simulink model "completed_microinverter_setup"  (R2022a)
settings: Solver=FixedStepDiscrete  StartTime=0.0  StopTime=2  FixedStep=Ts  RelTol=1e-3
InitFcn:
  | Ts=1e-6;
  | Tcs=1e-4;
values from neighbouring files (symbols this model uses):
  C1_filter = 2e-6    (= 2e-06)    [q4.m]
  C_filter = 100e-6    (= 0.0001)    [q1.m]    (also in q2.m; q4.m = 2e-06)
  f_center = 50    [q4.m]
  F_switch = 1e3    (= 1000)    [q1.m]
  Ki_current = L_filter*Wn^2    (= 15791.3670417)    [q1.m]    (also in q2.m = 63165.468167; q4.m = 493.480220054)
  Ki_pll = (Wn^2) / A    (= 394784.176044)    [q1.m]    (also in q4.m = 1579136.70417)
  Ki_power = 100    [q4.m]
  Ki_voltage = C_filter*Wn^2    (= 3.55305758439)    [q1.m]    (also in q4.m = 0.0710611516878)
  Kp_current = 2*L_filter*DF*Wn    (= 110.584061406)    [q1.m]    (also in q2.m = 71.0753921948; q4.m = 5.49778714378)
  Kp_pll = 2*DF / sqrt(A/Ki_pll)    [q1.m]    (also in q4.m = 2*DF / sqrt(1/Ki_pll))
  Kp_power = 0    [q4.m]
  Kp_voltage = 2*C_filter*DF*Wn    (= 0.0565486677646)    [q1.m]    (also in q4.m = 0.00791681348705)
  L1_filter = 1.5e-3    (= 0.0015)    [q4.m]
  L2_filter = 1.0e-3    (= 0.001)    [q4.m]
  L_filter = 40e-3    (= 0.04)    [q1.m]    (also in q2.m; q4.m = 0.00125)
  L_load = sqrt((R_load * V_rms^2)/P_load - R_load^2) / w    [q1.m]    (also in q4.m)
  R_load = (V_rms^2) * (pf_load^2) / P_load    (= 43.32)    [q1.m]    (also in q4.m)
  Rd_filter = 0.2    [q4.m]
  Tes = 20*Ts    (= 2e-05)    [q1.m]    (also in q4.m)
  V_dc = sqrt(2) * sqrt(3) * V_rms    [q1.m]    (also in q4.m = V_rms * sqrt(3) * sqrt(2))
undefined symbols (not defined in the file or in its folder): DiscIntNeverNeededParam
libraries: ee_lib x111, nesl_utility x28, fl_lib x23, spsabctodq0Lib x11, dspindex x3, spsTriangleGeneratorLib x2, spsdq0toabcLib x2
(part 2 of 4)

== system completed_microinverter_setup/Transmission line series impedance ==
  Inductor1 : ee_lib/Passive/Inductor  l=L H  enable_L_tol=0  L_tol=20  tol_distribution=1  nSigma=4  r=0 Ohm  g=1e-9 1/Ohm  enable_operating_limits=0  operating_limit_action=2  max_working_current=1 A  power_rating=1 W  enable_faults=0  fault_action=1  lambdaPercent=50  k_faulted=0.9999  turnsShort=0  openCct=0  groundShort=0  groundShortG=0 1/Ohm  tau_fault=1e-3 s  enable_temporal_fault=0  t_fault=1 s  enable_behavioral_fault=0  max_permissible_voltage=100 V  n_fail_on_voltage=1  max_permissible_current=1 A  t_fail_on_current=1 s  i_L_specify=off  i_L_priority=High  i_L=0 A  i_L_nominal_specify=off  i_L_nominal_unit=A  i_L_nominal_value=1
  Inductor2 : ee_lib/Passive/Inductor  l=L H  enable_L_tol=0  L_tol=20  tol_distribution=1  nSigma=4  r=0 Ohm  g=1e-9 1/Ohm  enable_operating_limits=0  operating_limit_action=2  max_working_current=1 A  power_rating=1 W  enable_faults=0  fault_action=1  lambdaPercent=50  k_faulted=0.9999  turnsShort=0  openCct=0  groundShort=0  groundShortG=0 1/Ohm  tau_fault=1e-3 s  enable_temporal_fault=0  t_fault=1 s  enable_behavioral_fault=0  max_permissible_voltage=100 V  n_fail_on_voltage=1  max_permissible_current=1 A  t_fail_on_current=1 s  i_L_specify=off  i_L_priority=High  i_L=0 A  i_L_nominal_specify=off  i_L_nominal_unit=A  i_L_nominal_value=1
  Inductor3 : ee_lib/Passive/Inductor  l=L H  enable_L_tol=0  L_tol=20  tol_distribution=1  nSigma=4  r=0 Ohm  g=1e-9 1/Ohm  enable_operating_limits=0  operating_limit_action=2  max_working_current=1 A  power_rating=1 W  enable_faults=0  fault_action=1  lambdaPercent=50  k_faulted=0.9999  turnsShort=0  openCct=0  groundShort=0  groundShortG=0 1/Ohm  tau_fault=1e-3 s  enable_temporal_fault=0  t_fault=1 s  enable_behavioral_fault=0  max_permissible_voltage=100 V  n_fail_on_voltage=1  max_permissible_current=1 A  t_fail_on_current=1 s  i_L_specify=off  i_L_priority=High  i_L=0 A  i_L_nominal_specify=off  i_L_nominal_unit=A  i_L_nominal_value=1
  Phase Splitter : ee_lib/Connectors & References/Phase Splitter
      settings: SourceProductBaseCode=PS
  Phase Splitter1 : ee_lib/Connectors & References/Phase Splitter
      settings: SourceProductBaseCode=PS
  Resistor : ee_lib/Passive/Resistor  R=R Ohm  enable_R_tol=0  R_tol=5  tol_distribution=1  nSigma=4  enable_operating_limits=0  operating_limit_action=2  max_working_voltage=100 V  power_rating=1 W  enable_faults=0  fault_action=1  R_faulted=inf Ohm  enable_temporal_fault=0  t_fault=1 s  enable_behavioral_fault=0  max_permissible_current=1 A  t_fail_on_current=1 s  noise_mode=0  sample_time=1e-3 s  repeatability=1  auto_seed=676943032  user_seed=0  Tdevice=25 degC  power_derating_T1=70 degC  power_derating_T2=155 degC  operating_temperature_range_vec=[-50, 150] degC  alpha=3.93e-3 1/K  Tmeas=25 degC  thermal_mass=100 J/K  temperature_specify=off  temperature_priority=High  temperature=298.15 K  temperature_nominal_specify=off  temperature_nominal_unit=K  temperature_nominal_value=1
  Resistor1 : ee_lib/Passive/Resistor  R=R Ohm  enable_R_tol=0  R_tol=5  tol_distribution=1  nSigma=4  enable_operating_limits=0  operating_limit_action=2  max_working_voltage=100 V  power_rating=1 W  enable_faults=0  fault_action=1  R_faulted=inf Ohm  enable_temporal_fault=0  t_fault=1 s  enable_behavioral_fault=0  max_permissible_current=1 A  t_fail_on_current=1 s  noise_mode=0  sample_time=1e-3 s  repeatability=1  auto_seed=4168664255  user_seed=0  Tdevice=25 degC  power_derating_T1=70 degC  power_derating_T2=155 degC  operating_temperature_range_vec=[-50, 150] degC  alpha=3.93e-3 1/K  Tmeas=25 degC  thermal_mass=100 J/K  temperature_specify=off  temperature_priority=High  temperature=298.15 K  temperature_nominal_specify=off  temperature_nominal_unit=K  temperature_nominal_value=1
  Resistor2 : ee_lib/Passive/Resistor  R=R Ohm  enable_R_tol=0  R_tol=5  tol_distribution=1  nSigma=4  enable_operating_limits=0  operating_limit_action=2  max_working_voltage=100 V  power_rating=1 W  enable_faults=0  fault_action=1  R_faulted=inf Ohm  enable_temporal_fault=0  t_fault=1 s  enable_behavioral_fault=0  max_permissible_current=1 A  t_fail_on_current=1 s  noise_mode=0  sample_time=1e-3 s  repeatability=1  auto_seed=4111000739  user_seed=0  Tdevice=25 degC  power_derating_T1=70 degC  power_derating_T2=155 degC  operating_temperature_range_vec=[-50, 150] degC  alpha=3.93e-3 1/K  Tmeas=25 degC  thermal_mass=100 J/K  temperature_specify=off  temperature_priority=High  temperature=298.15 K  temperature_nominal_specify=off  temperature_nominal_unit=K  temperature_nominal_value=1
  V_in : PMIOPort  Side=Left
  V_out : PMIOPort  Port=2  Side=Right
  connections:
  Phase Splitter1/RConn1 -- Inductor3/LConn1
  Inductor2/LConn1 -- Phase Splitter1/RConn3
  Inductor1/LConn1 -- Phase Splitter1/RConn2
  V_in/RConn1 -- Phase Splitter1/LConn1
  Resistor1/LConn1 -- Inductor1/RConn1
  Phase Splitter/RConn3 -- Resistor2/RConn1
  Phase Splitter/RConn1 -- Resistor/RConn1
  V_out/RConn1 -- Phase Splitter/LConn1
  Resistor/LConn1 -- Inductor3/RConn1
  Phase Splitter/RConn2 -- Resistor1/RConn1
  Resistor2/LConn1 -- Inductor2/RConn1

== system completed_microinverter_setup/Calculate PQ of output/Subsystem ==
  Vdq0 : Inport
  Constant : Constant
  Demux : Demux  Outputs=3
  Divide : Product  Inputs=*/
  Gain : Gain  Gain=-1
  Matrix Concatenate : Concatenate  Mode=Multidimensional array
  Matrix Concatenate1 : Concatenate  Mode=Multidimensional array  ConcatenateDimension=2
  Mux : Mux
  Reshape : Reshape  OutputDimensionality=Customize  OutputDimensions=[2,2]
  Sqrt1 : Sqrt
  Sqrt2 : Sqrt
  Square1 : Math  Operator=square
  Subtract : Sum  Inputs=+-
  Sum : Sum  Inputs=|++
  Terminator : Terminator
  Zero : Constant  Value=zeros(1,2)  VectorParams1D=off  OutDataTypeStr=Inherit: Inherit via back propagation
  Zero1 : Constant  Value=zeros(3,1)  VectorParams1D=off  OutDataTypeStr=Inherit: Inherit via back propagation
  Rotation Matrix : Outport
  wires:
  Vdq0/1 -> Square1/1
  Demux/1 -> Divide/1, Sum/1  "Vd^2"
  Reshape/1 -> Matrix Concatenate/1
  Gain/1 -> Mux/2
  Divide/1 -> Subtract/2, Sqrt1/1  "Vd^2 / (Vd^2 + Vq^2)"
  Sqrt2/1 -> Mux/3, Gain/1  "sin(theta)"
  Subtract/1 -> Sqrt2/1
  Demux/3 -> Terminator/1
  Square1/1 -> Demux/1
  Mux/1 -> Reshape/1
  Demux/2 -> Sum/2  "Vq^2"
  Constant/1 -> Subtract/1
  Sqrt1/1 -> Mux/4, Mux/1  "cos(theta)"
  Sum/1 -> Divide/2
  Zero/1 -> Matrix Concatenate/2
  Zero1/1 -> Matrix Concatenate1/2
  Matrix Concatenate/1 -> Matrix Concatenate1/1
  Matrix Concatenate1/1 -> Rotation Matrix/1

== system completed_microinverter_setup/Grid Feeding//Forming Inverter 1/3 Phase Grid Sensor ==
  Neutral Port (Three-Phase) : ee_lib/Connectors & References/Neutral Port (Three-Phase)  G_parasitic=1e-12 1/Ohm
      settings: SourceProductBaseCode=PS  InternalSimscapePortConfiguration="{\"Bottom\":[],\"Left\":[{\"id\":\"N\",\"label\":\"~\",\"type\":\"foundation.electrical.three_phase\"}],\"Right\":[{\"id\":\"n\",\"label\":\"n\",\"type\":\"foundation.electrical.electrical\"}],\"Top\":[]}"
  PS-Simulink Converter : nesl_utility/PS-Simulink Converter  PhysicalDomain=network_engine_domain  SubClassName=ps_output  LeftPortType=input  RightPortType=output  PseudoPeriodic=off  Frequencies=[]  VectorFormat=inherit  Unit=inherit  AffineConversion=off
      settings: SourceProductBaseCode=SS,PW,VE
  Phase Splitter1 : ee_lib/Connectors & References/Phase Splitter
      settings: SourceProductBaseCode=PS
  Phase Voltage Sensor (Three-Phase) : ee_lib/Sensors & Transducers/Phase Voltage Sensor (Three-Phase)
      settings: SourceProductBaseCode=PS
  Resistor : ee_lib/Passive/Resistor  R=R Ohm  enable_R_tol=0  R_tol=5  tol_distribution=1  nSigma=4  enable_operating_limits=0  operating_limit_action=2  max_working_voltage=100 V  power_rating=1 W  enable_faults=0  fault_action=1  R_faulted=inf Ohm  enable_temporal_fault=0  t_fault=1 s  enable_behavioral_fault=0  max_permissible_current=1 A  t_fail_on_current=1 s  noise_mode=0  sample_time=1e-3 s  repeatability=1  auto_seed=2715962282  user_seed=0  Tdevice=25 degC  power_derating_T1=70 degC  power_derating_T2=155 degC  operating_temperature_range_vec=[-50, 150] degC  alpha=3.93e-3 1/K  Tmeas=25 degC  thermal_mass=100 J/K  temperature_specify=off  temperature_priority=High  temperature=298.15 K  temperature_nominal_specify=off  temperature_nominal_unit=K  temperature_nominal_value=1
  Resistor1 : ee_lib/Passive/Resistor  R=R Ohm  enable_R_tol=0  R_tol=5  tol_distribution=1  nSigma=4  enable_operating_limits=0  operating_limit_action=2  max_working_voltage=100 V  power_rating=1 W  enable_faults=0  fault_action=1  R_faulted=inf Ohm  enable_temporal_fault=0  t_fault=1 s  enable_behavioral_fault=0  max_permissible_current=1 A  t_fail_on_current=1 s  noise_mode=0  sample_time=1e-3 s  repeatability=1  auto_seed=418932850  user_seed=0  Tdevice=25 degC  power_derating_T1=70 degC  power_derating_T2=155 degC  operating_temperature_range_vec=[-50, 150] degC  alpha=3.93e-3 1/K  Tmeas=25 degC  thermal_mass=100 J/K  temperature_specify=off  temperature_priority=High  temperature=298.15 K  temperature_nominal_specify=off  temperature_nominal_unit=K  temperature_nominal_value=1
  Resistor2 : ee_lib/Passive/Resistor  R=R Ohm  enable_R_tol=0  R_tol=5  tol_distribution=1  nSigma=4  enable_operating_limits=0  operating_limit_action=2  max_working_voltage=100 V  power_rating=1 W  enable_faults=0  fault_action=1  R_faulted=inf Ohm  enable_temporal_fault=0  t_fault=1 s  enable_behavioral_fault=0  max_permissible_current=1 A  t_fail_on_current=1 s  noise_mode=0  sample_time=1e-3 s  repeatability=1  auto_seed=1196140742  user_seed=0  Tdevice=25 degC  power_derating_T1=70 degC  power_derating_T2=155 degC  operating_temperature_range_vec=[-50, 150] degC  alpha=3.93e-3 1/K  Tmeas=25 degC  thermal_mass=100 J/K  temperature_specify=off  temperature_priority=High  temperature=298.15 K  temperature_nominal_specify=off  temperature_nominal_unit=K  temperature_nominal_value=1
  V_abc : PMIOPort  Side=Left
  V_abc_sense : Outport
  wires:
  PS-Simulink Converter/1 -> V_abc_sense/1
  connections:
  Resistor2/LConn1 -- Phase Splitter1/RConn3
  Resistor/RConn1 -- Neutral Port (Three-Phase)/RConn1 -- Resistor2/RConn1 -- Resistor1/RConn1
  Phase Splitter1/RConn2 -- Resistor1/LConn1
  Phase Splitter1/RConn1 -- Resistor/LConn1
  V_abc/RConn1 -- Phase Voltage Sensor (Three-Phase)/LConn1 -- Phase Splitter1/LConn1
  Phase Voltage Sensor (Three-Phase)/RConn2 -- Neutral Port (Three-Phase)/LConn1
  PS-Simulink Converter/LConn1 -- Phase Voltage Sensor (Three-Phase)/RConn1

== system completed_microinverter_setup/Grid Feeding//Forming Inverter 1/Calculate PQ of output ==
  note: Reorient Vdq0 so that Uq = 0, Ud = defined
  Vdq0 : Inport
  Idq0 : Inport  Port=2
  Atan2 : Trigonometry  Operator=atan2
  Cos : Trigonometry  Operator=cos
  Demux : Demux  Outputs=3
  Demux1 : Demux  Outputs=2
  Gain2 : Gain  Gain=3/2
  MatrixMultiply1 : Product  Multiplication=Matrix(*)
  MatrixMultiply2 : Product  Multiplication=Matrix(*)
  Mux : Mux
  Product : Product
  Product2 : Product
  Selector : Selector  InputPortWidth=3  IndexOptions=Index vector (dialog)  Indices=[1 2]  OutputSizes=1
  Selector1 : Selector  InputPortWidth=3  IndexOptions=Index vector (dialog)  Indices=[1]  OutputSizes=1
  Sign : Signum
  Sqrt : Sqrt
  Square : Math  Operator=square
  Subsystem : Subsystem
  Sum of Elements : Sum  Inputs=+
  Terminator : Terminator
  PQ Stats : Outport
  wires:
  Product2/1 -> Gain2/1
  Square/1 -> Sum of Elements/1
  Gain2/1 -> Demux/1, Selector/1
  Sum of Elements/1 -> Sqrt/1
  Selector/1 -> Square/1, Demux1/1
  Vdq0/1 -> MatrixMultiply1/2, Subsystem/1(Vdq0)
  Subsystem/1(Rotation Matrix) -> MatrixMultiply2/1, MatrixMultiply1/1
  Idq0/1 -> MatrixMultiply2/2
  MatrixMultiply1/1 -> Selector1/1
  MatrixMultiply2/1 -> Product2/2
  Demux/3 -> Terminator/1
  Demux/2 -> Atan2/1  "Q"
  Demux/1 -> Atan2/2  "P"
  Atan2/1 -> Cos/1
  Demux1/1 -> Mux/1  "P"
  Demux1/2 -> Sign/1, Mux/2  "Q"
  Sqrt/1 -> Mux/3  "|S|"
  Product/1 -> Mux/4  "pf"
  Mux/1 -> PQ Stats/1
  Selector1/1 -> Product2/1
  Sign/1 -> Product/1
  Cos/1 -> Product/2  "pf"

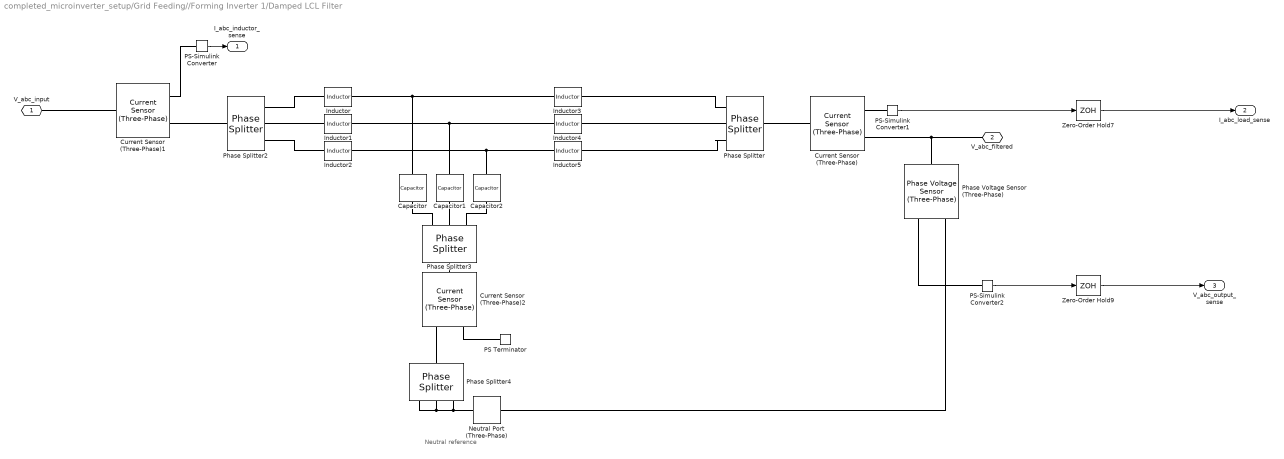
== system completed_microinverter_setup/Grid Feeding//Forming Inverter 1/Damped LCL Filter ==
  note: Neutral reference
  Capacitor : fl_lib/Electrical/Electrical Elements/Capacitor  c=C F  r=Rd Ohm  g=0 1/Ohm  i_specify=off  i_priority=None  i=0 A  i_nominal_specify=off  i_nominal_unit=A  i_nominal_value=1  v_specify=off  v_priority=None  v=0 V  v_nominal_specify=off  v_nominal_unit=V  v_nominal_value=1  vc_specify=off  vc_priority=High  vc=0 V  vc_nominal_specify=off  vc_nominal_unit=V  vc_nominal_value=1
      settings: SourceProductBaseCode=PW,SS,VE
  Capacitor1 : fl_lib/Electrical/Electrical Elements/Capacitor  c=C F  r=Rd Ohm  g=0 1/Ohm  i_specify=off  i_priority=None  i=0 A  i_nominal_specify=off  i_nominal_unit=A  i_nominal_value=1  v_specify=off  v_priority=None  v=0 V  v_nominal_specify=off  v_nominal_unit=V  v_nominal_value=1  vc_specify=off  vc_priority=High  vc=0 V  vc_nominal_specify=off  vc_nominal_unit=V  vc_nominal_value=1
      settings: SourceProductBaseCode=PW,SS,VE
  Capacitor2 : fl_lib/Electrical/Electrical Elements/Capacitor  c=C F  r=Rd Ohm  g=0 1/Ohm  i_specify=off  i_priority=None  i=0 A  i_nominal_specify=off  i_nominal_unit=A  i_nominal_value=1  v_specify=off  v_priority=None  v=0 V  v_nominal_specify=off  v_nominal_unit=V  v_nominal_value=1  vc_specify=off  vc_priority=High  vc=0 V  vc_nominal_specify=off  vc_nominal_unit=V  vc_nominal_value=1
      settings: SourceProductBaseCode=PW,SS,VE
  Current Sensor (Three-Phase) : ee_lib/Sensors & Transducers/Current Sensor (Three-Phase)
  Current Sensor (Three-Phase)1 : ee_lib/Sensors & Transducers/Current Sensor (Three-Phase)
  Current Sensor (Three-Phase)2 : ee_lib/Sensors & Transducers/Current Sensor (Three-Phase)
  Inductor : ee_lib/Passive/Inductor  l=L1 H  enable_L_tol=0  L_tol=20  tol_distribution=1  nSigma=4  r=0 Ohm  g=1e-9 1/Ohm  enable_operating_limits=0  operating_limit_action=2  max_working_current=1 A  power_rating=1 W  enable_faults=0  fault_action=1  lambdaPercent=50  k_faulted=0.9999  turnsShort=0  openCct=0  groundShort=0  groundShortG=0 1/Ohm  tau_fault=1e-3 s  enable_temporal_fault=0  t_fault=1 s  enable_behavioral_fault=0  max_permissible_voltage=100 V  n_fail_on_voltage=1  max_permissible_current=1 A  t_fail_on_current=1 s  i_L_specify=off  i_L_priority=High  i_L=0 A  i_L_nominal_specify=off  i_L_nominal_unit=A  i_L_nominal_value=1
  Inductor1 : ee_lib/Passive/Inductor  l=L1 H  enable_L_tol=0  L_tol=20  tol_distribution=1  nSigma=4  r=0 Ohm  g=1e-9 1/Ohm  enable_operating_limits=0  operating_limit_action=2  max_working_current=1 A  power_rating=1 W  enable_faults=0  fault_action=1  lambdaPercent=50  k_faulted=0.9999  turnsShort=0  openCct=0  groundShort=0  groundShortG=0 1/Ohm  tau_fault=1e-3 s  enable_temporal_fault=0  t_fault=1 s  enable_behavioral_fault=0  max_permissible_voltage=100 V  n_fail_on_voltage=1  max_permissible_current=1 A  t_fail_on_current=1 s  i_L_specify=off  i_L_priority=High  i_L=0 A  i_L_nominal_specify=off  i_L_nominal_unit=A  i_L_nominal_value=1
  Inductor2 : ee_lib/Passive/Inductor  l=L1 H  enable_L_tol=0  L_tol=20  tol_distribution=1  nSigma=4  r=0 Ohm  g=1e-9 1/Ohm  enable_operating_limits=0  operating_limit_action=2  max_working_current=1 A  power_rating=1 W  enable_faults=0  fault_action=1  lambdaPercent=50  k_faulted=0.9999  turnsShort=0  openCct=0  groundShort=0  groundShortG=0 1/Ohm  tau_fault=1e-3 s  enable_temporal_fault=0  t_fault=1 s  enable_behavioral_fault=0  max_permissible_voltage=100 V  n_fail_on_voltage=1  max_permissible_current=1 A  t_fail_on_current=1 s  i_L_specify=off  i_L_priority=High  i_L=0 A  i_L_nominal_specify=off  i_L_nominal_unit=A  i_L_nominal_value=1
  Inductor3 : ee_lib/Passive/Inductor  l=L2 H  enable_L_tol=0  L_tol=20  tol_distribution=1  nSigma=4  r=0 Ohm  g=1e-9 1/Ohm  enable_operating_limits=0  operating_limit_action=2  max_working_current=1 A  power_rating=1 W  enable_faults=0  fault_action=1  lambdaPercent=50  k_faulted=0.9999  turnsShort=0  openCct=0  groundShort=0  groundShortG=0 1/Ohm  tau_fault=1e-3 s  enable_temporal_fault=0  t_fault=1 s  enable_behavioral_fault=0  max_permissible_voltage=100 V  n_fail_on_voltage=1  max_permissible_current=1 A  t_fail_on_current=1 s  i_L_specify=off  i_L_priority=High  i_L=0 A  i_L_nominal_specify=off  i_L_nominal_unit=A  i_L_nominal_value=1
  Inductor4 : ee_lib/Passive/Inductor  l=L2 H  enable_L_tol=0  L_tol=20  tol_distribution=1  nSigma=4  r=0 Ohm  g=1e-9 1/Ohm  enable_operating_limits=0  operating_limit_action=2  max_working_current=1 A  power_rating=1 W  enable_faults=0  fault_action=1  lambdaPercent=50  k_faulted=0.9999  turnsShort=0  openCct=0  groundShort=0  groundShortG=0 1/Ohm  tau_fault=1e-3 s  enable_temporal_fault=0  t_fault=1 s  enable_behavioral_fault=0  max_permissible_voltage=100 V  n_fail_on_voltage=1  max_permissible_current=1 A  t_fail_on_current=1 s  i_L_specify=off  i_L_priority=High  i_L=0 A  i_L_nominal_specify=off  i_L_nominal_unit=A  i_L_nominal_value=1
  Inductor5 : ee_lib/Passive/Inductor  l=L2 H  enable_L_tol=0  L_tol=20  tol_distribution=1  nSigma=4  r=0 Ohm  g=1e-9 1/Ohm  enable_operating_limits=0  operating_limit_action=2  max_working_current=1 A  power_rating=1 W  enable_faults=0  fault_action=1  lambdaPercent=50  k_faulted=0.9999  turnsShort=0  openCct=0  groundShort=0  groundShortG=0 1/Ohm  tau_fault=1e-3 s  enable_temporal_fault=0  t_fault=1 s  enable_behavioral_fault=0  max_permissible_voltage=100 V  n_fail_on_voltage=1  max_permissible_current=1 A  t_fail_on_current=1 s  i_L_specify=off  i_L_priority=High  i_L=0 A  i_L_nominal_specify=off  i_L_nominal_unit=A  i_L_nominal_value=1
  Neutral Port (Three-Phase) : ee_lib/Connectors & References/Neutral Port (Three-Phase)  G_parasitic=1e-12 1/Ohm
      settings: SourceProductBaseCode=PS  InternalSimscapePortConfiguration="{\"Bottom\":[],\"Left\":[{\"id\":\"N\",\"label\":\"~\",\"type\":\"foundation.electrical.three_phase\"}],\"Right\":[{\"id\":\"n\",\"label\":\"n\",\"type\":\"foundation.electrical.electrical\"}],\"Top\":[]}"
  PS Terminator : fl_lib/Physical Signals/Sinks/PS Terminator
      settings: SourceProductBaseCode=PW,SS,VE
  PS-Simulink Converter : nesl_utility/PS-Simulink Converter  PhysicalDomain=network_engine_domain  SubClassName=ps_output  LeftPortType=input  RightPortType=output  PseudoPeriodic=off  Frequencies=[]  VectorFormat=inherit  Unit=inherit  AffineConversion=off
      settings: SourceProductBaseCode=SS,PW,VE
  PS-Simulink Converter1 : nesl_utility/PS-Simulink Converter  PhysicalDomain=network_engine_domain  SubClassName=ps_output  LeftPortType=input  RightPortType=output  PseudoPeriodic=off  Frequencies=[]  VectorFormat=inherit  Unit=inherit  AffineConversion=off
      settings: SourceProductBaseCode=SS,PW,VE
  PS-Simulink Converter2 : nesl_utility/PS-Simulink Converter  PhysicalDomain=network_engine_domain  SubClassName=ps_output  LeftPortType=input  RightPortType=output  PseudoPeriodic=off  Frequencies=[]  VectorFormat=inherit  Unit=inherit  AffineConversion=off
      settings: SourceProductBaseCode=SS,PW,VE
  Phase Splitter{,2..4} (4 alike) : ee_lib/Connectors & References/Phase Splitter
      settings: SourceProductBaseCode=PS
  Phase Voltage Sensor (Three-Phase) : ee_lib/Sensors & Transducers/Phase Voltage Sensor (Three-Phase)
      settings: SourceProductBaseCode=PS
  Zero-Order Hold7 : ZeroOrderHold  SampleTime=Ts
  Zero-Order Hold9 : ZeroOrderHold  SampleTime=Ts
  V_abc_input : PMIOPort  Side=Left
  V_abc_filtered : PMIOPort  Port=2  Side=Right
  I_abc_inductor_sense : Outport
  I_abc_load_sense : Outport  Port=2
  V_abc_output_sense : Outport  Port=3
  wires:
  PS-Simulink Converter/1 -> I_abc_inductor_sense/1
  PS-Simulink Converter1/1 -> Zero-Order Hold7/1
  Zero-Order Hold7/1 -> I_abc_load_sense/1
  PS-Simulink Converter2/1 -> Zero-Order Hold9/1
  Zero-Order Hold9/1 -> V_abc_output_sense/1
  connections:
  Capacitor1/LConn1 -- Inductor4/LConn1 -- Inductor1/RConn1
  Capacitor/LConn1 -- Inductor3/LConn1 -- Inductor/RConn1
  Capacitor2/LConn1 -- Inductor5/LConn1 -- Inductor2/RConn1
  Phase Voltage Sensor (Three-Phase)/LConn1 -- Current Sensor (Three-Phase)/RConn2 -- V_abc_filtered/RConn1
  Phase Voltage Sensor (Three-Phase)/RConn2 -- Neutral Port (Three-Phase)/LConn1
  Current Sensor (Three-Phase)/LConn1 -- Phase Splitter/LConn1
  Phase Splitter2/RConn2 -- Inductor1/LConn1
  Phase Splitter2/RConn1 -- Inductor/LConn1
  Phase Splitter2/RConn3 -- Inductor2/LConn1
  Phase Splitter2/LConn1 -- Current Sensor (Three-Phase)1/RConn2
  PS-Simulink Converter/LConn1 -- Current Sensor (Three-Phase)1/RConn1
  PS-Simulink Converter1/LConn1 -- Current Sensor (Three-Phase)/RConn1
  PS-Simulink Converter2/LConn1 -- Phase Voltage Sensor (Three-Phase)/RConn1
  Phase Splitter3/RConn1 -- Capacitor/RConn1
  Phase Splitter3/RConn2 -- Capacitor1/RConn1
  Phase Splitter3/RConn3 -- Capacitor2/RConn1
  Phase Splitter3/LConn1 -- Current Sensor (Three-Phase)2/LConn1
  Phase Splitter4/LConn1 -- Current Sensor (Three-Phase)2/RConn2
  Phase Splitter4/RConn1 -- Neutral Port (Three-Phase)/RConn1 -- Phase Splitter4/RConn3 -- Phase Splitter4/RConn2
  V_abc_input/RConn1 -- Current Sensor (Three-Phase)1/LConn1
  Phase Splitter/RConn1 -- Inductor3/RConn1
  Phase Splitter/RConn2 -- Inductor4/RConn1
  Phase Splitter/RConn3 -- Inductor5/RConn1
  PS Terminator/LConn1 -- Current Sensor (Three-Phase)2/RConn1

== system completed_microinverter_setup/Grid Feeding//Forming Inverter 1/Ideal Inverter ==
  U_abc_control : Inport
  Controlled Voltage Source : fl_lib/Electrical/Electrical Sources/Controlled Voltage Source
      settings: SourceProductBaseCode=PW,SS,VE
  Controlled Voltage Source1 : fl_lib/Electrical/Electrical Sources/Controlled Voltage Source
      settings: SourceProductBaseCode=PW,SS,VE
  Controlled Voltage Source2 : fl_lib/Electrical/Electrical Sources/Controlled Voltage Source
      settings: SourceProductBaseCode=PW,SS,VE
  Delay : Delay  DelayLength=1
  Demux : Demux  Outputs=3
  Electrical Reference : fl_lib/Electrical/Electrical Elements/Electrical Reference
      settings: SourceProductBaseCode=PW,SS,VE
  Phase Splitter : ee_lib/Connectors & References/Phase Splitter
      settings: SourceProductBaseCode=PS
  Simulink-PS Converter3 : nesl_utility/Simulink-PS Converter  PhysicalDomain=network_engine_domain  SubClassName=ps_input  LeftPortType=input  RightPortType=output  PseudoPeriodic=off  Frequencies=[]  NoiseDistribution=none  NoiseParameters=[]  Unit=1  AffineConversion=off  FilteringAndDerivatives=provide  SimscapeFilterOrder=1  InputFilterTimeConstant=0.001  UdotUserProvided=0
      settings: SourceProductBaseCode=SS,PW,VE
  Simulink-PS Converter4 : nesl_utility/Simulink-PS Converter  PhysicalDomain=network_engine_domain  SubClassName=ps_input  LeftPortType=input  RightPortType=output  PseudoPeriodic=off  Frequencies=[]  NoiseDistribution=none  NoiseParameters=[]  Unit=1  AffineConversion=off  FilteringAndDerivatives=provide  SimscapeFilterOrder=1  InputFilterTimeConstant=0.001  UdotUserProvided=0
      settings: SourceProductBaseCode=SS,PW,VE
  Simulink-PS Converter5 : nesl_utility/Simulink-PS Converter  PhysicalDomain=network_engine_domain  SubClassName=ps_input  LeftPortType=input  RightPortType=output  PseudoPeriodic=off  Frequencies=[]  NoiseDistribution=none  NoiseParameters=[]  Unit=1  AffineConversion=off  FilteringAndDerivatives=provide  SimscapeFilterOrder=1  InputFilterTimeConstant=0.001  UdotUserProvided=0
      settings: SourceProductBaseCode=SS,PW,VE
  Zero-Order Hold6 : ZeroOrderHold  SampleTime=Tcs
  V_abc_out : PMIOPort  Side=Right
  wires:
  Demux/1 -> Simulink-PS Converter3/1
  Demux/2 -> Simulink-PS Converter4/1
  Demux/3 -> Simulink-PS Converter5/1
  Zero-Order Hold6/1 -> Delay/1
  Delay/1 -> Demux/1
  U_abc_control/1 -> Zero-Order Hold6/1
  connections:
  Phase Splitter/RConn1 -- Controlled Voltage Source/LConn1
  Phase Splitter/RConn3 -- Controlled Voltage Source2/LConn1
  Simulink-PS Converter5/RConn1 -- Controlled Voltage Source2/RConn1
  Electrical Reference/LConn1 -- Controlled Voltage Source/RConn2 -- Controlled Voltage Source1/RConn2 -- Controlled Voltage Source2/RConn2
  Phase Splitter/RConn2 -- Controlled Voltage Source1/LConn1
  Simulink-PS Converter3/RConn1 -- Controlled Voltage Source/RConn1
  Simulink-PS Converter4/RConn1 -- Controlled Voltage Source1/RConn1
  Phase Splitter/LConn1 -- V_abc_out/RConn1

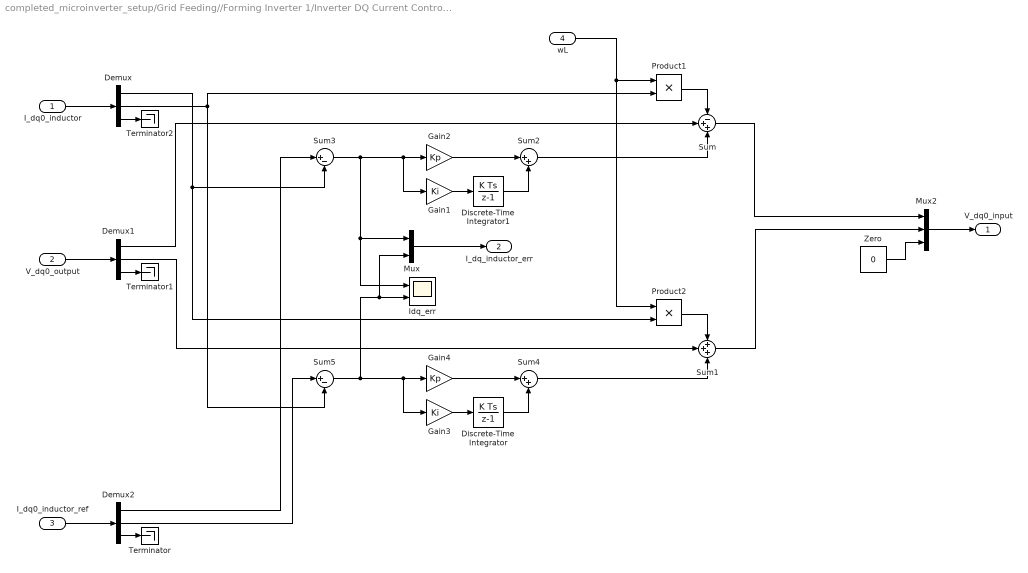
== system completed_microinverter_setup/Grid Feeding//Forming Inverter 1/Inverter DQ Current Controller ==
  I_dq0_inductor : Inport
  V_dq0_output : Inport  Port=2
  I_dq0_inductor_ref : Inport  Port=3
  wL : Inport  Port=4
  Demux : Demux  Outputs=3
  Demux1 : Demux  Outputs=3
  Demux2 : Demux  Outputs=3
  Discrete-Time Integrator : DiscreteIntegrator  SampleTime=Ts  ICPrevOutput=DiscIntNeverNeededParam  ICPrevScaledInput=DiscIntNeverNeededParam
  Discrete-Time Integrator1 : DiscreteIntegrator  SampleTime=Ts  ICPrevOutput=DiscIntNeverNeededParam  ICPrevScaledInput=DiscIntNeverNeededParam
  Gain1 : Gain  Gain=Ki
  Gain2 : Gain  Gain=Kp
  Gain3 : Gain  Gain=Ki
  Gain4 : Gain  Gain=Kp
  Idq_err : Scope  NumInputPorts=2
  Mux : Mux  Inputs=2
  Mux2 : Mux  Inputs=3
  Product1 : Product
  Product2 : Product
  Sum : Sum  Inputs=-++
  Sum1 : Sum  Inputs=+++
  Sum2 : Sum  Inputs=|++
  Sum3 : Sum  Inputs=|+-
  Sum4 : Sum  Inputs=|++
  Sum5 : Sum  Inputs=|+-
  Terminator : Terminator
  Terminator1 : Terminator
  Terminator2 : Terminator
  Zero : Constant  Value=0  OutDataTypeStr=Inherit: Inherit via back propagation
  V_dq0_input : Outport
  I_dq_inductor_err : Outport  Port=2
  wires:
  Gain3/1 -> Discrete-Time Integrator/1
  I_dq0_inductor_ref/1 -> Demux2/1
  V_dq0_output/1 -> Demux1/1
  Demux2/1 -> Sum3/1
  Discrete-Time Integrator1/1 -> Sum2/2
  Gain4/1 -> Sum4/1
  Product2/1 -> Sum1/1
  Sum5/1 -> Mux/2, Idq_err/2, Gain4/1, Gain3/1
  Mux2/1 -> V_dq0_input/1
  Demux/2 -> Sum5/2, Product1/2
  Demux/1 -> Sum3/2, Product2/2
  Demux2/3 -> Terminator/1
  I_dq0_inductor/1 -> Demux/1
  Sum/1 -> Mux2/1
  Demux1/1 -> Sum/2
  Discrete-Time Integrator/1 -> Sum4/2
  Product1/1 -> Sum/1
  Gain2/1 -> Sum2/1
  Sum2/1 -> Sum/3
  Gain1/1 -> Discrete-Time Integrator1/1
  Sum1/1 -> Mux2/2
  Zero/1 -> Mux2/3
  Sum4/1 -> Sum1/3
  Demux1/2 -> Sum1/2
  Demux2/2 -> Sum5/1
  Demux1/3 -> Terminator1/1
  Demux/3 -> Terminator2/1
  wL/1 -> Product2/1, Product1/1
  Sum3/1 -> Mux/1, Idq_err/1, Gain2/1, Gain1/1
  Mux/1 -> I_dq_inductor_err/1

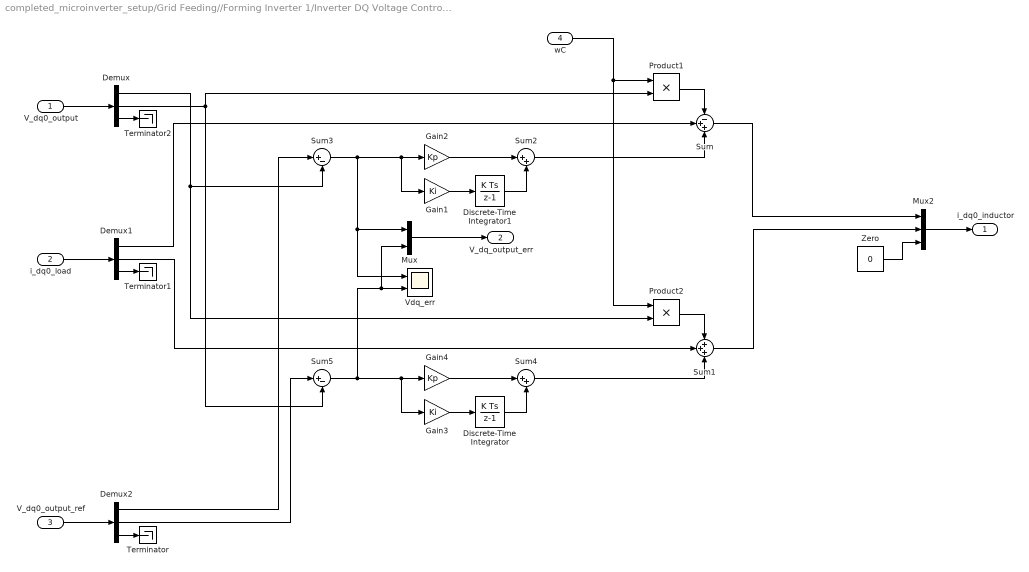
== system completed_microinverter_setup/Grid Feeding//Forming Inverter 1/Inverter DQ Voltage Controller ==
  V_dq0_output : Inport
  i_dq0_load : Inport  Port=2
  V_dq0_output_ref : Inport  Port=3
  wC : Inport  Port=4
  Demux : Demux  Outputs=3
  Demux1 : Demux  Outputs=3
  Demux2 : Demux  Outputs=3
  Discrete-Time Integrator : DiscreteIntegrator  SampleTime=Ts  ICPrevOutput=DiscIntNeverNeededParam  ICPrevScaledInput=DiscIntNeverNeededParam
  Discrete-Time Integrator1 : DiscreteIntegrator  SampleTime=Ts  ICPrevOutput=DiscIntNeverNeededParam  ICPrevScaledInput=DiscIntNeverNeededParam
  Gain1 : Gain  Gain=Ki
  Gain2 : Gain  Gain=Kp
  Gain3 : Gain  Gain=Ki
  Gain4 : Gain  Gain=Kp
  Mux : Mux  Inputs=2
  Mux2 : Mux  Inputs=3
  Product1 : Product
  Product2 : Product
  Sum : Sum  Inputs=-++
  Sum1 : Sum  Inputs=+++
  Sum2 : Sum  Inputs=|++
  Sum3 : Sum  Inputs=|+-
  Sum4 : Sum  Inputs=|++
  Sum5 : Sum  Inputs=|+-
  Terminator : Terminator
  Terminator1 : Terminator
  Terminator2 : Terminator
  Vdq_err : Scope  NumInputPorts=2
  Zero : Constant  Value=0  OutDataTypeStr=Inherit: Inherit via back propagation
  i_dq0_inductor : Outport
  V_dq_output_err : Outport  Port=2
  wires:
  Gain3/1 -> Discrete-Time Integrator/1
  V_dq0_output_ref/1 -> Demux2/1
  i_dq0_load/1 -> Demux1/1
  Demux2/1 -> Sum3/1
  Discrete-Time Integrator1/1 -> Sum2/2
  Gain4/1 -> Sum4/1
  Product2/1 -> Sum1/1
  Sum5/1 -> Mux/2, Vdq_err/2, Gain4/1, Gain3/1
  Mux2/1 -> i_dq0_inductor/1
  Demux/2 -> Sum5/2, Product1/2
  Demux/1 -> Sum3/2, Product2/2
  Sum3/1 -> Mux/1, Vdq_err/1, Gain2/1, Gain1/1
  Demux2/3 -> Terminator/1
  V_dq0_output/1 -> Demux/1
  Sum/1 -> Mux2/1
  Demux1/1 -> Sum/2
  Discrete-Time Integrator/1 -> Sum4/2
  Product1/1 -> Sum/1
  Gain2/1 -> Sum2/1
  Sum2/1 -> Sum/3
  Gain1/1 -> Discrete-Time Integrator1/1
  Sum1/1 -> Mux2/2
  Zero/1 -> Mux2/3
  Sum4/1 -> Sum1/3
  Demux1/2 -> Sum1/2
  Demux2/2 -> Sum5/1
  Demux1/3 -> Terminator1/1
  Demux/3 -> Terminator2/1
  wC/1 -> Product2/1, Product1/1
  Mux/1 -> V_dq_output_err/1

== system completed_microinverter_setup/Grid Feeding//Forming Inverter 1/Inverter PI Power Controller ==
  note: Load current PI controller
  note: Use a feedforward term since we know that
      | Idq0_inductor = Idq0_load + Idq0_capacitor
      |
      | We let Idq0_capacitor be compensated for by the integrator
  note: Don't integrate error when operating in grid forming mode
  note: P-Q to Idq0_load conversion
  note: P=Vrms * Irms cos(theta)
      | P = 1/2 * VI * cos(theta)
      |
      | Since Id = Icos(theta), when locked onto V (the output/grid voltage)
      | V = Vd (When PLL is locked onto the grid)
      |
      | P = 1/2 * Vd * Id
      |
      | Since we have 3 phases
      | P = 3/2 * Vd * Id
      |
      | Therefore for a reference power, we get
      | Id_ref = P * 2/3 * (1/Vd)
      |
      | Likewise for Q = Vrms * Irms * sin(theta)
      | Iq_ref = Q * 2/3 * (1/Vd)
  P_ref : Inport
  Q_ref : Inport  Port=2
  Vd : Inport  Port=3
  I_dq0_load_in : Inport  Port=4
  Grid Connect Signal : Inport  Port=5
  Constant11 : Constant  Value=0
  Demux1 : Demux  Outputs=2
  Discrete-Time Integrator2 : DiscreteIntegrator  SampleTime=Ts  LimitOutput=on  UpperSaturationLimit=100  LowerSaturationLimit=-100  ICPrevOutput=DiscIntNeverNeededParam  ICPrevScaledInput=DiscIntNeverNeededParam
  Divide : Product  Inputs=*/
  Gain1 : Gain  Gain=2/3
  Gain2 : Gain  Gain=Kp
  Gain4 : Gain  Gain=Ki
  Mux : Mux  Inputs=2
  Mux3 : Mux  Inputs=3
  Scope : Scope
  Scope7 : Scope
  Scope9 : Scope  NumInputPorts=2
  Sum : Sum  Inputs=+-|
  Sum1 : Sum  Inputs=|++
  Sum2 : Sum  Inputs=|++
  Switch1 : Switch  Criteria=u2 > Threshold  SaturateOnIntegerOverflow=off  InputSameDT=off
  Zero : Constant  Value=0  OutDataTypeStr=Inherit: Inherit via back propagation
  I_dq0_inductor : Outport
  wires:
  Sum/1 -> Switch1/1  "I_dq0_error"
  Zero/1 -> Switch1/3
  Discrete-Time Integrator2/1 -> Sum1/2
  Sum2/1 -> I_dq0_inductor/1
  Gain4/1 -> Discrete-Time Integrator2/1
  Grid Connect Signal/1 -> Switch1/2
  Gain1/1 -> Divide/1
  Demux1/1 -> Mux3/1  "Id"
  Constant11/1 -> Mux3/3
  Demux1/2 -> Mux3/2  "Iq"
  Divide/1 -> Demux1/1
  Q_ref/1 -> Mux/2
  P_ref/1 -> Mux/1
  Vd/1 -> Divide/2
  Mux/1 -> Gain1/1
  Mux3/1 -> Scope9/1, Sum/1, Sum2/1  "I_dq0_load_ref"
  Switch1/1 -> Scope7/1, Gain4/1, Gain2/1
  Gain2/1 -> Sum1/1
  Sum1/1 -> Scope/1, Sum2/2  "I_dq0_adjust"
  I_dq0_load_in/1 -> Scope9/2, Sum/2

== system completed_microinverter_setup/Grid Feeding//Forming Inverter 1/PLL ==
  Vabc : Inport
  Constant1 : Constant  Value=f_center  SampleTime=-1
  Delay : Delay  DelayLength=1  SampleTime=Ts
  Demux : Demux  Outputs=3
  Divide : Product  Inputs=*/
  Gain : Gain  Gain=2*pi
  Gain3 : Gain  Gain=2/3
  PI Controller : Subsystem
  Saturation : Saturate  UpperLimit=2*pi*4.8  LowerLimit=-2*pi*4.8
  Scope{,2..4} (4 alike) : Scope
  Sqrt : Sqrt
  Square : Math  Operator=square
  Sum of Elements : Sum  Inputs=+
  Terminator : Terminator
  Terminator1 : Terminator
  Transform : Subsystem
  Zero-Order Hold : ZeroOrderHold  SampleTime=Ts
  abc to dq0 : spsabctodq0Lib/abc to dq0  Alignment=Aligned with phase A axis
  Amp_est : Outport
  w_est : Outport  Port=2
  wt : Outport  Port=3
  Vdq0 : Outport  Port=4
  wires:
  Square/1 -> Sum of Elements/1
  Sum of Elements/1 -> Gain3/1
  Gain3/1 -> Sqrt/1
  Constant1/1 -> Transform/2(f_center)
  Divide/1 -> PI Controller/1(Vq)
  PI Controller/1(U) -> Saturation/1
  Sqrt/1 -> Divide/2, Scope/1, Amp_est/1
  Transform/2(f_out) -> Scope2/1, Gain/1
  Transform/1(wt) -> abc to dq0/2, wt/1
  Zero-Order Hold/1 -> Scope4/1, abc to dq0/1, Square/1
  Saturation/1 -> Delay/1
  Delay/1 -> Transform/1(U)
  Vabc/1 -> Zero-Order Hold/1
  abc to dq0/1 -> Scope3/1, Vdq0/1, Demux/1
  Demux/2 -> Divide/1
  Gain/1 -> w_est/1
  Demux/3 -> Terminator/1
  Demux/1 -> Terminator1/1
